simulink model "decoder_3x8"  (R2015a)
settings: Solver=ode45  StartTime=0.0  StopTime=10.0  RelTol=1e-3
settings Model: Creator=citd  LastModifiedBy=citd

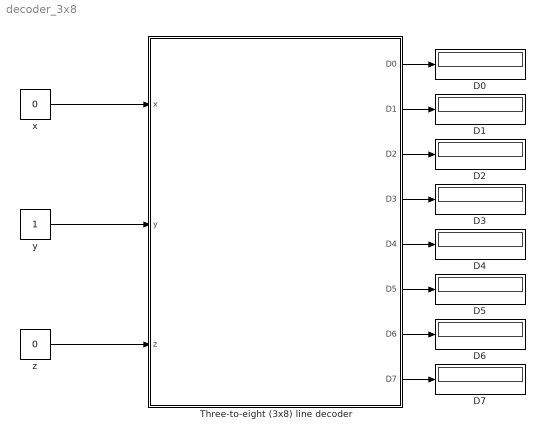
== system decoder_3x8 ==
  D{0..7} (8 alike) : Display
  Three-to-eight (3x8) line decoder : Subsystem
  x : Constant  Value=0  OutDataTypeStr=boolean
  y : Constant  OutDataTypeStr=boolean
  z : Constant  Value=0  OutDataTypeStr=boolean
  wires:
  z/1 -> Three-to-eight (3x8) line decoder/3(z)
  x/1 -> Three-to-eight (3x8) line decoder/1(x)
  y/1 -> Three-to-eight (3x8) line decoder/2(y)
  Three-to-eight (3x8) line decoder/1(D0) -> D0/1
  Three-to-eight (3x8) line decoder/2(D1) -> D1/1
  Three-to-eight (3x8) line decoder/3(D2) -> D2/1
  Three-to-eight (3x8) line decoder/4(D3) -> D3/1
  Three-to-eight (3x8) line decoder/5(D4) -> D4/1
  Three-to-eight (3x8) line decoder/6(D5) -> D5/1
  Three-to-eight (3x8) line decoder/7(D6) -> D6/1
  Three-to-eight (3x8) line decoder/8(D7) -> D7/1

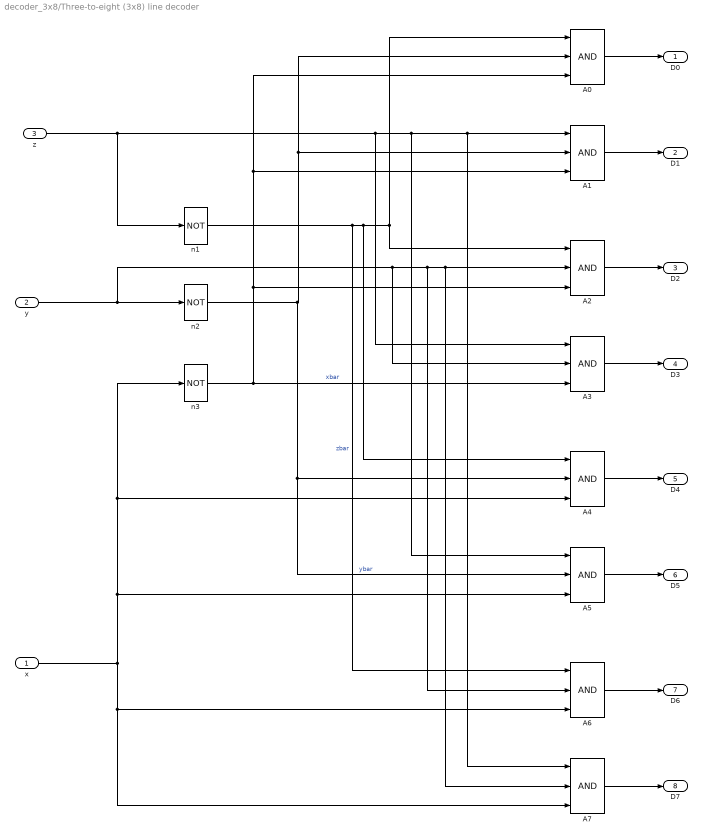
== system decoder_3x8/Three-to-eight (3x8) line decoder ==
  x : Inport
  y : Inport  Port=2
  z : Inport  Port=3
  A{0..7} (8 alike) : Logic  Inputs=3  IconShape=distinctive  AllPortsSameDT=off  OutDataTypeStr=boolean
  n1 : Logic  Operator=NOT  Inputs=3  IconShape=distinctive  AllPortsSameDT=off  OutDataTypeStr=boolean
  n2 : Logic  Operator=NOT  Inputs=3  IconShape=distinctive  AllPortsSameDT=off  OutDataTypeStr=boolean
  n3 : Logic  Operator=NOT  Inputs=3  IconShape=distinctive  AllPortsSameDT=off  OutDataTypeStr=boolean
  D0 : Outport
  D1 : Outport  Port=2
  D2 : Outport  Port=3
  D3 : Outport  Port=4
  D4 : Outport  Port=5
  D5 : Outport  Port=6
  D6 : Outport  Port=7
  D7 : Outport  Port=8
  wires:
  A6/1 -> D6/1
  A1/1 -> D1/1
  A2/1 -> D2/1
  A5/1 -> D5/1
  A4/1 -> D4/1
  A7/1 -> D7/1
  A3/1 -> D3/1
  A0/1 -> D0/1
  y/1 -> n2/1, A2/2, A7/2, A6/2, A3/2
  x/1 -> A6/3, A7/3, A5/3, A4/3, n3/1
  z/1 -> A1/1, A7/1, A5/1, A3/1, n1/1
  n2/1 -> A0/2, A1/2, A4/2, A5/2  "ybar"
  n3/1 -> A3/3, A0/3, A1/3, A2/3  "xbar"
  n1/1 -> A2/1, A0/1, A4/1, A6/1  "zbar"
